simulink model "lin_model"  (R2019a)
settings: Solver=VariableStepAuto  StartTime=0.0  StopTime=10  RelTol=1e-3
values from neighbouring files (symbols this model uses):
  g = 9.80665    [drone.m]    (also in step-af-drone.m = -150*(1+0.001*s)/s)
undefined symbols (not defined in the file or in its folder): Ix, Iy, Iz, l, m
settings Model: Creator=Hillerup  LastModifiedBy=Hillerup

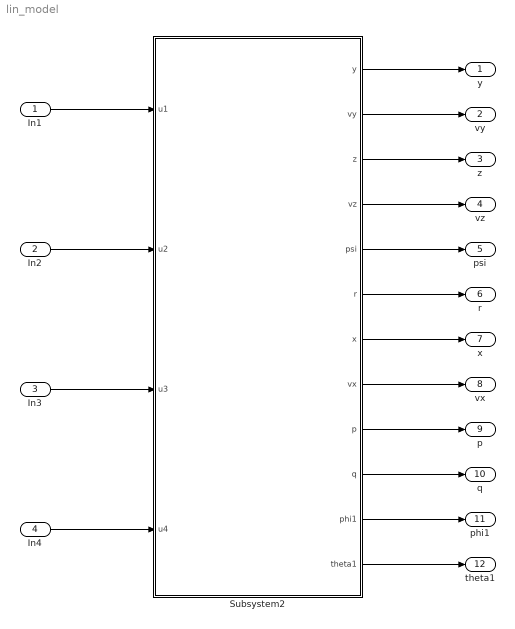
== system lin_model ==
  In1 : Inport
  In2 : Inport  Port=2
  In3 : Inport  Port=3
  In4 : Inport  Port=4
  Subsystem2 : Subsystem
  y : Outport
  vy : Outport  Port=2
  z : Outport  Port=3
  vz : Outport  Port=4
  psi : Outport  Port=5
  r : Outport  Port=6
  "x " : Outport  Port=7
  vx : Outport  Port=8
  p : Outport  Port=9
  q : Outport  Port=10
  phi1 : Outport  Port=11
  theta1 : Outport  Port=12
  wires:
  Subsystem2/1(y) -> y/1
  Subsystem2/2(vy) -> vy/1
  Subsystem2/4(vz) -> vz/1
  Subsystem2/5(psi) -> psi/1
  Subsystem2/6(r) -> r/1
  Subsystem2/8(vx) -> vx/1
  Subsystem2/9(p) -> p/1
  Subsystem2/10(q) -> q/1
  Subsystem2/11(phi1) -> phi1/1
  Subsystem2/12(theta1) -> theta1/1
  Subsystem2/3(z) -> z/1
  Subsystem2/7("x ") -> "x "/1
  In1/1 -> Subsystem2/1(u1)
  In2/1 -> Subsystem2/2(u2)
  In3/1 -> Subsystem2/3(u3)
  In4/1 -> Subsystem2/4(u4)

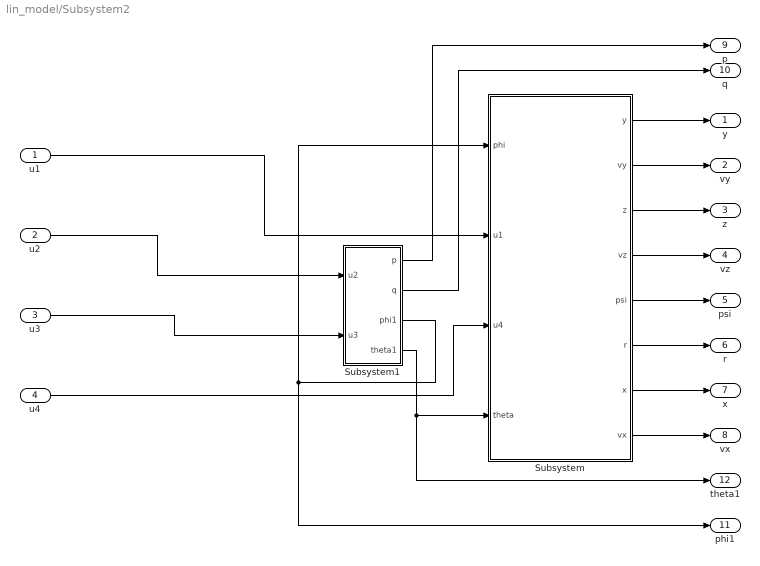
== system lin_model/Subsystem2 ==
  u1 : Inport
  u2 : Inport  Port=2
  u3 : Inport  Port=3
  u4 : Inport  Port=4
  Subsystem : Subsystem
  Subsystem1 : Subsystem
  y : Outport
  vy : Outport  Port=2
  z : Outport  Port=3
  vz : Outport  Port=4
  psi : Outport  Port=5
  r : Outport  Port=6
  "x " : Outport  Port=7
  vx : Outport  Port=8
  p : Outport  Port=9
  q : Outport  Port=10
  phi1 : Outport  Port=11
  theta1 : Outport  Port=12
  wires:
  Subsystem/3(z) -> z/1
  Subsystem/2(vy) -> vy/1
  Subsystem/1(y) -> y/1
  Subsystem1/2(q) -> q/1
  Subsystem1/3(phi1) -> Subsystem/1(phi), phi1/1
  Subsystem/6(r) -> r/1
  Subsystem1/4(theta1) -> theta1/1, Subsystem/4(theta)
  Subsystem/7("x ") -> "x "/1
  Subsystem/4(vz) -> vz/1
  Subsystem/5(psi) -> psi/1
  Subsystem/8(vx) -> vx/1
  Subsystem1/1(p) -> p/1
  u3/1 -> Subsystem1/2(u3)
  u2/1 -> Subsystem1/1(u2)
  u4/1 -> Subsystem/3(u4)
  u1/1 -> Subsystem/2(u1)

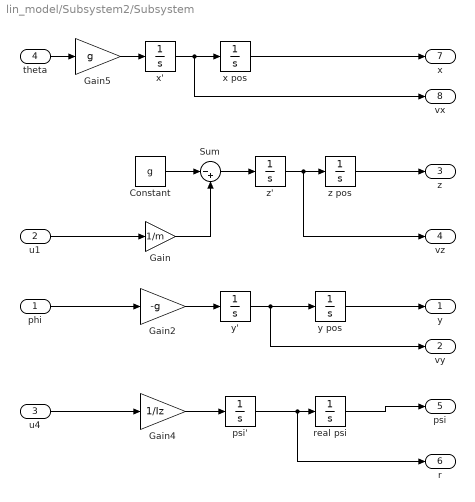
== system lin_model/Subsystem2/Subsystem ==
  phi : Inport
  u1 : Inport  Port=2
  u4 : Inport  Port=3  OutDataTypeStr=double
  theta : Inport  Port=4
  Constant : Constant  Value=g
  Gain : Gain  Gain=1/m
  Gain2 : Gain  Gain=-g
  Gain4 : Gain  Gain=1/Iz  OutDataTypeStr=double
  Gain5 : Gain  Gain=g
  Sum : Sum  Inputs=|-+
  psi' : Integrator
  real psi : Integrator
  x pos : Integrator
  x' : Integrator
  y pos : Integrator
  y' : Integrator
  z pos : Integrator
  z' : Integrator
  y : Outport
  vy : Outport  Port=2
  z : Outport  Port=3
  vz : Outport  Port=4
  psi : Outport  Port=5  OutDataTypeStr=double
  r : Outport  Port=6  OutDataTypeStr=double
  "x " : Outport  Port=7
  vx : Outport  Port=8
  wires:
  theta/1 -> Gain5/1
  psi'/1 -> r/1, real psi/1
  z'/1 -> vz/1, z pos/1
  x pos/1 -> "x "/1
  x'/1 -> vx/1, x pos/1
  Gain2/1 -> y'/1
  Gain5/1 -> x'/1
  phi/1 -> Gain2/1
  Constant/1 -> Sum/1
  z pos/1 -> z/1
  Gain/1 -> Sum/2
  u1/1 -> Gain/1
  real psi/1 -> psi/1
  u4/1 -> Gain4/1
  y'/1 -> vy/1, y pos/1
  y pos/1 -> y/1
  Sum/1 -> z'/1
  Gain4/1 -> psi'/1

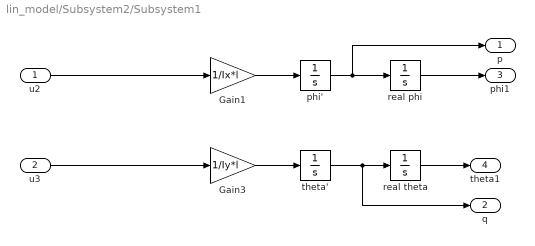
== system lin_model/Subsystem2/Subsystem1 ==
  u2 : Inport
  u3 : Inport  Port=2
  Gain1 : Gain  Gain=1/Ix*l
  Gain3 : Gain  Gain=1/Iy*l
  phi' : Integrator
  real phi : Integrator
  real theta : Integrator
  theta' : Integrator
  p : Outport
  q : Outport  Port=2
  phi1 : Outport  Port=3
  theta1 : Outport  Port=4
  wires:
  Gain3/1 -> theta'/1
  Gain1/1 -> phi'/1
  theta'/1 -> q/1, real theta/1
  phi'/1 -> p/1, real phi/1
  real theta/1 -> theta1/1
  u3/1 -> Gain3/1
  real phi/1 -> phi1/1
  u2/1 -> Gain1/1
